simulink model "fz6_8"  (R2014a)
settings: Solver=ode45  StartTime=0.0  StopTime=10.0  RelTol=1e-3
libraries: commutil2 x4, commsink2 x2, commdigbbndam3 x2, commchan3 x1, commrandsrc2 x1
settings Model: Creator=tzb  LastModifiedBy=tzb

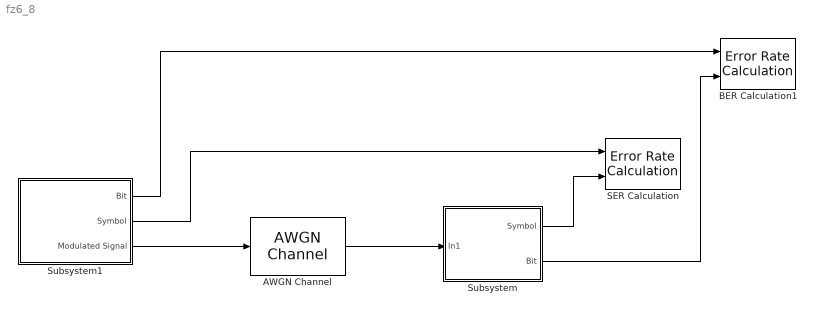
== system fz6_8 ==
  AWGN Channel : commchan3/AWGN Channel  InputProcessing=Columns as channels (frame based)  seed=67  noiseMode="Signal to noise ratio  (Es/No)"  EbNodB=10  EsNodB=SNR  SNRdB=10  bitsPerSym=1  Ps=5  Tsym=1/100000  variance=1
  BER Calculation1 : commsink2/Error Rate Calculation  N=0  st_delay=0  cp_mode=Entire frame  subframe=[]  PMode=Workspace  WsName=BER  RsMode2=off  stop=off  numErr=100  maxBits=1e6
  SER Calculation : commsink2/Error Rate Calculation  N=0  st_delay=0  cp_mode=Entire frame  subframe=[]  PMode=Workspace  WsName=SER  RsMode2=off  stop=off  numErr=100  maxBits=1e6
  Subsystem : Subsystem
  Subsystem1 : Subsystem
  wires:
  Subsystem1/3(Modulated Signal) -> AWGN Channel/1
  AWGN Channel/1 -> Subsystem/1(In1)
  Subsystem/1(Symbol) -> SER Calculation/2
  Subsystem/2(Bit) -> BER Calculation1/2
  Subsystem1/2(Symbol) -> SER Calculation/1
  Subsystem1/1(Bit) -> BER Calculation1/1

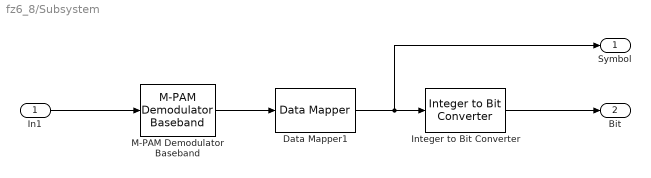
== system fz6_8/Subsystem ==
  In1 : Inport
  Data Mapper1 : commutil2/Data Mapper  MapMode=Binary to Gray  M=4  MapVec=[0 1 3 2 7 6 4 5]
  Integer to Bit Converter : commutil2/Integer to Bit Converter  nbits=2  signedInputValues=Unsigned  bitOrder=MSB first  outDtype=Inherit via internal rule
  M-PAM Demodulator Baseband : commdigbbndam3/M-PAM Demodulator Baseband  M=4  OutType=Integer  Dec=Gray  PowType=Min. distance between symbols  MinDist=2  AvgPow=1  PeakPow=1  outDtype1=Inherit via internal rule  outDtype2=Inherit via internal rule  denormFactorWordLen=16  prodOutWordLen=16  prodOutRoundingMode=Floor  prodOutOverflowMode=Wrap  sumWordLen=16
  Symbol : Outport
  Bit : Outport  Port=2
  wires:
  Integer to Bit Converter/1 -> Bit/1
  In1/1 -> M-PAM Demodulator Baseband/1
  M-PAM Demodulator Baseband/1 -> Data Mapper1/1
  Data Mapper1/1 -> Symbol/1, Integer to Bit Converter/1

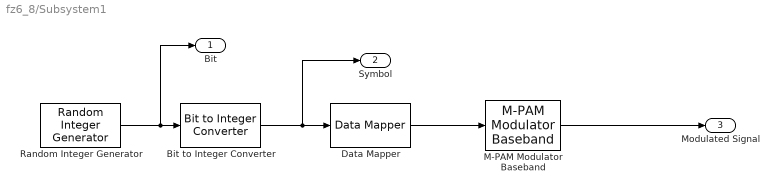
== system fz6_8/Subsystem1 ==
  Bit to Integer Converter : commutil2/Bit to Integer Converter  nbits=2  bitOrder=MSB first  signedOutputValues=Unsigned  outDtype=Inherit via internal rule  outDtypeSigned=Inherit via internal rule
  Data Mapper : commutil2/Data Mapper  MapMode=Binary to Gray  M=4  MapVec=[0 1 3 2 7 6 4 5]
  M-PAM Modulator Baseband : commdigbbndam3/M-PAM Modulator Baseband  M=4  InType=Integer  Enc=Gray  PowType=Min. distance between symbols  MinDist=2  AvgPow=1  PeakPow=1  outDtype=double  outWordLen=16  outUDDataType=sfix(16)  outFracLenMode=Best precision  outFracLen=15
  Random Integer Generator : commrandsrc2/Random Integer Generator  mul=2  seed=37  Ts=1/200000  frameBased=on  sampPerFrame=200000  orient=off  outDataType=double
  Bit : Outport
  Symbol : Outport  Port=2
  Modulated Signal : Outport  Port=3
  wires:
  Bit to Integer Converter/1 -> Symbol/1, Data Mapper/1
  Data Mapper/1 -> M-PAM Modulator Baseband/1
  M-PAM Modulator Baseband/1 -> Modulated Signal/1
  Random Integer Generator/1 -> Bit/1, Bit to Integer Converter/1
